simulink model "fuzzypid"  (R2018b)
settings: Solver=VariableStepAuto  StartTime=0.0  StopTime=50  RelTol=1e-3
values from neighbouring files (symbols this model uses):
  xcos = 0:10    [variables.m]
  ycos = 0:10    [variables.m]
libraries: fuzblock x2, simulink x2
settings Model: Creator=axelwillekens  LastModifiedBy=axelwillekens

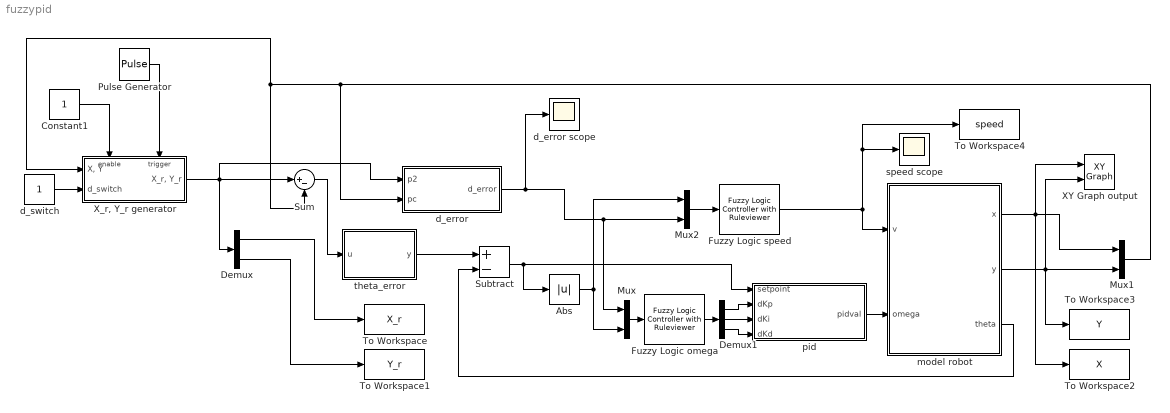
== system fuzzypid ==
  Abs : Abs
  Constant1 : Constant
  Demux : Demux  Outputs=2
  Demux1 : Demux  Outputs=3
  Fuzzy Logic omega : fuzblock/Fuzzy Logic  Controller  with Ruleviewer  fismatrix=fisomega  Ts=2
  Fuzzy Logic speed : fuzblock/Fuzzy Logic  Controller  with Ruleviewer  fismatrix=fisspeed  Ts=2
  Mux : Mux  Inputs=2
  Mux1 : Mux  Inputs=2
  Mux2 : Mux  Inputs=2
  Pulse Generator : DiscretePulseGenerator  PulseType=Time based  Period=0.05  PulseWidth=5
  Subtract : Sum  Inputs=+-
  Sum : Sum  Inputs=|+-
  To Workspace : ToWorkspace  VariableName=X_r  SaveFormat=Timeseries  SampleTime=-1
  To Workspace1 : ToWorkspace  VariableName=Y_r  SaveFormat=Timeseries  SampleTime=-1
  To Workspace2 : ToWorkspace  VariableName=X  SaveFormat=Timeseries  SampleTime=-1
  To Workspace3 : ToWorkspace  VariableName=Y  SaveFormat=Timeseries  SampleTime=-1
  To Workspace4 : ToWorkspace  VariableName=speed  SaveFormat=Timeseries  SampleTime=-1
  XY Graph output : simulink/Sinks/XY Graph  xmin=-2  xmax=50  ymin=-2  ymax=50  st=-1
  "X_r, Y_r generator" : Subsystem  TreatAsAtomicUnit=on
  d_error : MATLAB Function  TreatAsAtomicUnit=on
  d_error scope : Scope
  d_switch : Constant
  model robot : Subsystem
  pid : Subsystem
  speed scope : Scope
  theta_error : MATLAB Function  TreatAsAtomicUnit=on
  wires:
  Sum/1 -> theta_error/1(u)
  model robot/1(x) -> XY Graph output/1, To Workspace2/1, Mux1/1
  theta_error/1(y) -> Subtract/1
  Constant1/1 -> "X_r, Y_r generator"/Enable
  model robot/3(theta) -> Subtract/2
  Pulse Generator/1 -> "X_r, Y_r generator"/Trigger
  model robot/2(y) -> XY Graph output/2, To Workspace3/1, Mux1/2
  Demux/1 -> To Workspace/1
  d_switch/1 -> "X_r, Y_r generator"/2(d_switch)
  Fuzzy Logic speed/1 -> model robot/1(v), To Workspace4/1, speed scope/1
  pid/1(pidval) -> model robot/2(omega)
  Subtract/1 -> Abs/1, pid/1(setpoint)
  Demux1/1 -> pid/2(dKp)
  Demux1/2 -> pid/3(dKi)
  Demux1/3 -> pid/4(dKd)
  Fuzzy Logic omega/1 -> Demux1/1
  Mux/1 -> Fuzzy Logic omega/1
  Abs/1 -> Mux/2, Mux2/1
  d_error/1(d_error) -> Mux/1, Mux2/2, d_error scope/1
  Mux1/1 -> "X_r, Y_r generator"/1("X, Y"), Sum/2, d_error/2(pc)
  "X_r, Y_r generator"/1("X_r, Y_r") -> Demux/1, d_error/1(p2), Sum/1
  Mux2/1 -> Fuzzy Logic speed/1
  Demux/2 -> To Workspace1/1

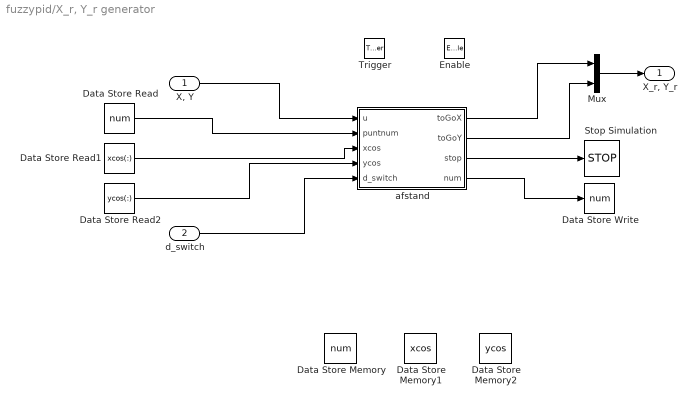
== system fuzzypid/X_r, Y_r generator ==
  "X, Y" : Inport
  d_switch : Inport  Port=2
  Enable : EnablePort
  Trigger : TriggerPort  VariantControl=Variant
  Data Store Memory : DataStoreMemory  DataStoreName=num  ReadBeforeWriteMsg=warning  WriteAfterWriteMsg=warning  WriteAfterReadMsg=warning  InitialValue=1  ShowAdditionalParam=off
  Data Store Memory1 : DataStoreMemory  DataStoreName=xcos  ReadBeforeWriteMsg=warning  WriteAfterWriteMsg=warning  WriteAfterReadMsg=warning  InitialValue=linspace(0,50,51)  ShowAdditionalParam=off
  Data Store Memory2 : DataStoreMemory  DataStoreName=ycos  ReadBeforeWriteMsg=warning  WriteAfterWriteMsg=warning  WriteAfterReadMsg=warning  InitialValue=linspace(0,50,51)  ShowAdditionalParam=off
  Data Store Read : DataStoreRead  DataStoreName=num  DataStoreElements=num
  Data Store Read1 : DataStoreRead  DataStoreName=xcos  DataStoreElements=xcos(:)
  Data Store Read2 : DataStoreRead  DataStoreName=ycos  DataStoreElements=ycos(:)
  Data Store Write : DataStoreWrite  DataStoreName=num  DataStoreElements=num
  Mux : Mux  Inputs=2
  Stop Simulation : Stop
  afstand : MATLAB Function  TreatAsAtomicUnit=on
  "X_r, Y_r" : Outport
  wires:
  "X, Y"/1 -> afstand/1(u)
  afstand/1(toGoX) -> Mux/1
  afstand/3(stop) -> Stop Simulation/1
  Data Store Read/1 -> afstand/2(puntnum)
  afstand/4(num) -> Data Store Write/1
  Data Store Read1/1 -> afstand/3(xcos)
  Data Store Read2/1 -> afstand/4(ycos)
  afstand/2(toGoY) -> Mux/2
  Mux/1 -> "X_r, Y_r"/1
  d_switch/1 -> afstand/5(d_switch)

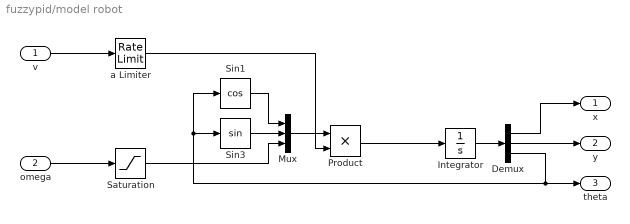
== system fuzzypid/model robot ==
  v : Inport
  omega : Inport  Port=2
  Demux : Demux  Outputs=3
  Integrator : Integrator  InitialCondition=[-1.5 -1 3*pi/4]
  Mux : Mux  Inputs=3
  Product : Product
  Saturation : Saturate  UpperLimit=1.2  LowerLimit=-1.2
  Sin1 : Trigonometry  Operator=cos
  Sin3 : Trigonometry
  a Limiter : RateLimiter  SampleTimeMode=inherited
  x : Outport
  y : Outport  Port=2
  theta : Outport  Port=3
  wires:
  v/1 -> a Limiter/1
  Mux/1 -> Product/1
  Product/1 -> Integrator/1
  Integrator/1 -> Demux/1
  Demux/2 -> y/1
  Demux/1 -> x/1
  Demux/3 -> Sin1/1, Sin3/1, theta/1
  Sin1/1 -> Mux/1
  omega/1 -> Saturation/1
  Sin3/1 -> Mux/2
  a Limiter/1 -> Product/2
  Saturation/1 -> Mux/3

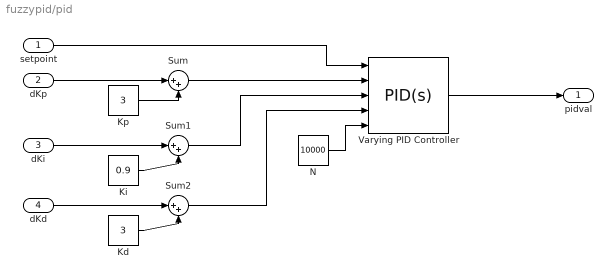
== system fuzzypid/pid ==
  setpoint : Inport
  dKp : Inport  Port=2
  dKi : Inport  Port=3
  dKd : Inport  Port=4
  Kd : Constant  Value=3
  Ki : Constant  Value=0.9
  Kp : Constant  Value=3
  N : Constant  Value=10000
  Sum : Sum  Inputs=|++
  Sum1 : Sum  Inputs=|++
  Sum2 : Sum  Inputs=|++
  Varying PID Controller : simulink/Continuous/PID Controller  Controller=PID  Form=Parallel  TimeDomain=Continuous-time  SampleTime=-1  IntegratorMethod=Forward Euler  FilterMethod=Forward Euler  ControllerParametersSource=external  P=1  I=1  D=0  UseFilter=on  N=100  TunerSelectOption=Transfer Function Based (PID Tuner App)  InitialConditionSource=internal  InitialConditionForIntegrator=0  InitialConditionForFilter=0  DifferentiatorICPrevScaledInput=0  ExternalReset=none  TrackingMode=off  Kt=1  LimitOutput=off  UpperSaturationLimit=inf  LowerSaturationLimit=-inf  LinearizeAsGain=on  AntiWindupMode=none  Kb=1  POutMin=[]  POutMax=[]  IOutMin=[]  IOutMax=[]  DOutMin=[]  DOutMax=[]  NOutMin=[]  NOutMax=[]  SumOutMin=[]  SumOutMax=[]  SaturationOutMin=[]  SaturationOutMax=[]  PParamMin=[]  PParamMax=[]  IParamMin=[]  IParamMax=[]  DParamMin=[]  DParamMax=[]  NParamMin=[]  NParamMax=[]  KbParamMin=[]  KbParamMax=[]  KtParamMin=[]  KtParamMax=[]  KbOutMin=[]  KbOutMax=[]  KtOutMin=[]  KtOutMax=[]  IntegratorOutMin=[]  IntegratorOutMax=[]  FilterOutMin=[]  FilterOutMax=[]  SumI1OutMin=[]  SumI1OutMax=[]  SumI2OutMin=[]  SumI2OutMax=[]  SumI3OutMin=[]  SumI3OutMax=[]  SumI4OutMin=[]  SumI4OutMax=[]  SumDOutMin=[]  SumDOutMax=[]  DifferentiatorOutMin=[]  DifferentiatorOutMax=[]  FilterDiffOutCoefMin=[]  FilterDiffOutCoefMax=[]  ReciprocalOutMin=[]  ReciprocalOutMax=[]  SumDenOutMin=[]  SumDenOutMax=[]  SumNumOutMin=[]  SumNumOutMax=[]  DivideOutMin=[]  DivideOutMax=[]  IntegratorContinuousStateAttributes=''  IntegratorStateMustResolveToSignalObject=off  IntegratorRTWStateStorageClass=Auto  FilterContinuousStateAttributes=''  FilterStateMustResolveToSignalObject=off  FilterRTWStateStorageClass=Auto  ParallelPVariant=ExternalParameters  IdealPVariant=Disabled  IVariant=ExternalParameters  DVariant=ExternalParameters  IntegratorVariant=Continuous  SatVariant=Disabled  AWVariant=Passthrough  PCopyVariant=Disabled  TRVariant=Disabled  FdbkBlocksVariant=Forward  IdealPFdbkVariant=Disabled  SatFdbkVariant=Disabled  DerivativeFilterVariant=ContFilter  NVariant=ExternalParameters  NCopyVariant=Disabled  FilterICVariant=InternalICsFilter  IntegratorICVariant=InternalICs  ExternalResetVariant=Disabled  TRSumVariant=Passthrough  SumFdbkVariant=Disabled  SumVariant=Sum_PID
  pidval : Outport
  wires:
  dKp/1 -> Sum/1
  dKi/1 -> Sum1/1
  dKd/1 -> Sum2/1
  Kp/1 -> Sum/2
  Ki/1 -> Sum1/2
  Kd/1 -> Sum2/2
  Sum/1 -> Varying PID Controller/2
  Sum1/1 -> Varying PID Controller/3
  Sum2/1 -> Varying PID Controller/4
  Varying PID Controller/1 -> pidval/1
  N/1 -> Varying PID Controller/5
  setpoint/1 -> Varying PID Controller/1

== matlab function fuzzypid/d_error ==
  settings: updateMethod=DISCRETE
  data: p2 input; pc input; d_error output
function d_error = fcn(p2, pc)
persistent p1 temp
if isempty(p1)
    p1 = [0; 0];
    temp = p1;
end

if temp ~= p2
    p1 = temp;
end
    
x1 = p1(1);
y1 = p1(2);
x2 = p2(1);
y2 = p2(2);
xc = pc(1);
yc = pc(2);

r = (y2 - y1)/(x2 - x1);
x = (yc + r*xc + r*x1 - y1)/(2*r);
y = r*x + (-r*x1 + y1);

temp = p2;
d_error = sqrt((xc - x)^2 + (yc - y)^2);

== matlab function fuzzypid/theta_error ==
  data: u input; y output
function y = fcn(u)

y = atan2(u(2),u(1));

== matlab function fuzzypid/X_r, Y_r generator/afstand ==
  data: u input; toGoX output; toGoY output; stop output; puntnum input; num output; xcos input; ycos input; d_switch input
function [toGoX, toGoY, stop, num] = fcn(u, puntnum, xcos, ycos, d_switch)
d = sqrt((xcos(puntnum)-u(1))^2 + (ycos(puntnum)-u(2))^2);
if d < d_switch
    num = puntnum + 1;
else
    num = puntnum;
end

toGoX = xcos(puntnum); 
toGoY = ycos(puntnum);

if num > length(xcos)
    stop = 1;
else
    stop = 0;
end
